simulink model "TwoQuadrantDCDCConverter"  (R2024a)
settings: Solver=VariableStepAuto  StartTime=0.0  StopTime=0.03  MaxStep=1e-4  RelTol=1e-4  EnableMultiTasking=on
libraries: spsGroundLib x3, spsDCVoltageSourceLib x2, spsSeriesRLCBranchLib x2, spsMeanLib x2, spsCurrentMeasurementLib x1, spsVoltageMeasurementLib x1, spsPWMGeneratorDCDCLib x1, spsTwoQuadrantDCDCConverterLib x1, sps_lib x1
settings Model: Creator=The MathWorks, Inc.  LastModifiedBy=nakamura
settings SolverCC: AlgebraicLoopSolver=TrustRegion  SolverResetMethod=Robust
settings OptimizationCC: LifeSpan=inf
settings DebuggingCC: ReadBeforeWriteMsg=DisableAll  WriteAfterWriteMsg=DisableAll  WriteAfterReadMsg=DisableAll  MultiTaskDSMMsg=none  UnconnectedInputMsg=warning  UnconnectedOutputMsg=warning  UnconnectedLineMsg=warning  SFUnexpectedBacktrackingDiag=warning  SFNoUnconditionalDefaultTransitionDiag=warning  SFExecutionAtInitializationDiag=none  ArithmeticOperatorsInVariantConditions=warning
settings ModelReferenceCC: UpdateModelReferenceTargets=IfOutOfDate  EnableRefExpFcnMdlSchedulingChecks=on
settings SFSimCC: SFSimEcho=off  SimUseLocalCustomCode=off  CustomCodeUndefinedFunction=UseInterfaceOnly
settings RTWCC: RTWUseLocalCustomCode=off  GPUComputeCapability=3.5
settings CodeAppCC: StateflowObjectComments=on
settings GRTTargetCC: TargetLangStandard=C89/C90 (ANSI)
settings ConfigComp: CovMetricSettings=dw  CovSaveCumulativeToWorkspaceVar=on  CovSaveSingleToWorkspaceVar=on  CovExternalEMLEnable=off
settings SimscapeCC: SimscapeNormalizeSystem=off  SimscapeNominalValues={1, 'bar'; 1, 'cm^3/s'; 1, 'bar*kg/s'; 1, 'kJ/kg'; 1, 'kW'; }

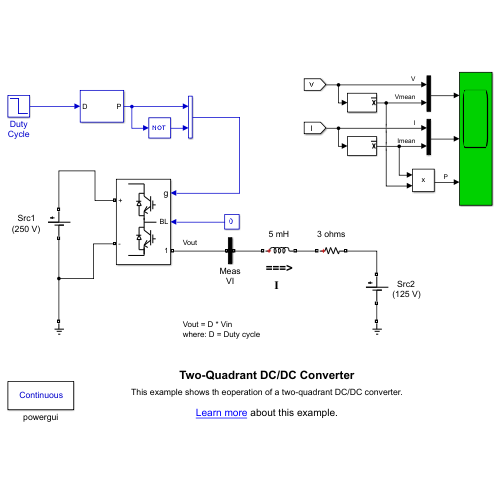
[thumbnail: Simulink's stored preview of the top-level diagram]
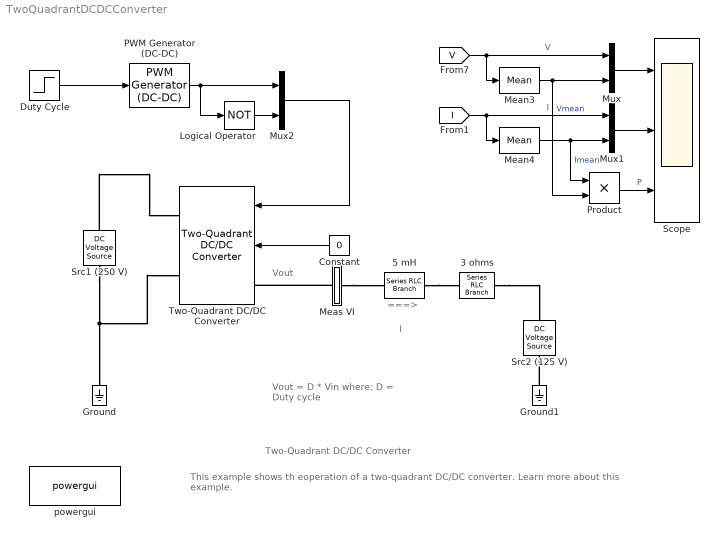
== system TwoQuadrantDCDCConverter ==
  note: Vout
  note: Vout = D * Vin
      | where: D = Duty cycle
  note: ===>
  note: I
  note: Two-Quadrant DC/DC Converter
  note: This example shows th eoperation of a two-quadrant DC/DC converter.
      |
      | Learn more about this example.
  "  Src2 (125 V)" : spsDCVoltageSourceLib/DC Voltage Source  Amplitude=125  Measurements=None
  3 ohms : spsSeriesRLCBranchLib/Series RLC Branch  LConnTagsString=__new0  RConnTagsString=__new0  BranchType=R  Resistance=3  Inductance=750e-6  SetiL0=on  InitialCurrent=14  Capacitance=30e-6  Setx0=off  InitialVoltage=150  Measurements=None
  5 mH : spsSeriesRLCBranchLib/Series RLC Branch  LConnTagsString=__new0  RConnTagsString=__new0  BranchType=L  Resistance=1e-4  Inductance=5e-3  SetiL0=off  InitialCurrent=14  Capacitance=30e-6  Setx0=off  InitialVoltage=150  Measurements=None
  Constant : Constant  Value=0
  Duty Cycle : Step  Time=0.015  Before=0.75  After=0.25  SampleTime=0
  Ground : spsGroundLib/Ground  LConnTagsString=a
  Ground1 : spsGroundLib/Ground  LConnTagsString=a
  Logical Operator : Logic  Operator=NOT  AllPortsSameDT=off  OutDataTypeStr=float('double')
  Mean3 : spsMeanLib/Mean  Freq=1000  Vinit=0  Ts=0
  Mean4 : spsMeanLib/Mean  Freq=1000  Vinit=0  Ts=0
  Meas VI : Subsystem
  Mux : Mux  Inputs=2
  Mux1 : Mux  Inputs=2
  Mux2 : Mux  Inputs=2
  PWM Generator (DC-DC) : spsPWMGeneratorDCDCLib/PWM Generator (DC-DC)  Fsw=2e3  Ts=0
  Product : Product
  Scope : Scope  NumInputPorts=3
  "Src1 (250 V) " : spsDCVoltageSourceLib/DC Voltage Source  Amplitude=250  Measurements=None
  Two-Quadrant DC/DC Converter : spsTwoQuadrantDCDCConverterLib/Two-Quadrant DC//DC Converter  ModelType=Switching devices  Ron=1e-3  Rs=1e6  Cs=inf  Vforward=[0,0]  Ron_Diode=1e-3  Rs_Diode=1e6  Cs_Diode=inf  Vf_Diode=1e-3  Rs_CurrentSource=inf  Ron_ACsource=1e-3
      settings: LibrarySourceBlock=|
      | sps_lib/Power Electronics/Two-Quadrant
      | DC//DC Converter
  powergui : sps_lib/powergui  Priority=1  SimulationMode=Continuous  SampleTime=1e-6  frequency=60  Iterations=50  frequencyindice=0  Pbase=100e6  ErrMax=1e-4  UnitsV=kV  UnitsW=MW  buscounter=0  FunctionMessages=off  echomessages=off  EnableUseOfTLC=off  CurrentSourceSwitches=off  DisableSnubberDevices=off  DisableRonSwitches=off  DisableVfSwitches=off  DisplayEquations=off  AutomaticDiscreteSolvers=off  SolverType=Tustin/Backward Euler (TBE)  Interpol=off  ExternalGateDelay=off  methode=off  Ts=100  x0status=blocks  SPID=on  SwTol=0  HookPort=off  NonlinearTolerance=1e-4  nMaxIteration=100  ContinueOnMaxIteration=off  RestoreLinks=warning  ResistiveCurrentMeasurement=off  Frange=[0:2:500]  Ylog=off  Xlog=on  ShowGrid=off  save=off  variable=ZData  structure=0  ZoomFFT=off  StartTime=0.0  cycles=1  DisplayStyle=1  fundamental=60  FreqAxis=off  MaxFrequency=1000  frequencyindicesteady=1  RmsSteady=1  display=off
  wires:
  Duty Cycle/1 -> PWM Generator (DC-DC)/1
  [V] -> Mean3/1, Mux/1  "V"
  Mux/1 -> Scope/1
  PWM Generator (DC-DC)/1 -> Logical Operator/1, Mux2/1
  Logical Operator/1 -> Mux2/2
  Constant/1 -> Two-Quadrant DC/DC Converter/2
  Mux2/1 -> Two-Quadrant DC/DC Converter/1
  Mean3/1 -> Product/2, Mux/2  "Vmean"
  [I] -> Mux1/1, Mean4/1  "I"
  Mean4/1 -> Product/1, Mux1/2  "Imean"
  Mux1/1 -> Scope/2
  Product/1 -> Scope/3  "P"
  connections:
  5 mH/RConn1 -- 3 ohms/LConn1
  3 ohms/RConn1 -- "  Src2 (125 V)"/RConn1
  "Src1 (250 V) "/RConn1 -- Two-Quadrant DC/DC Converter/RConn1
  "Src1 (250 V) "/LConn1 -- Two-Quadrant DC/DC Converter/RConn2 -- Ground/LConn1
  Meas VI/LConn1 -- Two-Quadrant DC/DC Converter/LConn1
  Meas VI/RConn1 -- 5 mH/LConn1
  Ground1/LConn1 -- "  Src2 (125 V)"/LConn1

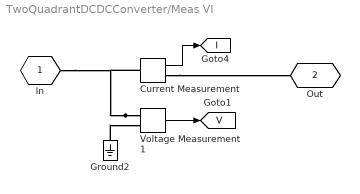
== system TwoQuadrantDCDCConverter/Meas VI ==
  Current Measurement : spsCurrentMeasurementLib/Current Measurement  PhasorSimulation=off  OutputType=Complex  PSBequivalent=0
  Ground2 : spsGroundLib/Ground  LConnTagsString=a
  Voltage Measurement1 : spsVoltageMeasurementLib/Voltage Measurement  Tag=PoWeRsYsTeMmEaSuReMeNt  PhasorSimulation=off  OutputType=Magnitude  PSBequivalent=0
  In : PMIOPort  Tag=PMCPort  Side=Left
  Out : PMIOPort  Tag=PMCPort  Port=2  Side=Right
  tag scope: I=global, V=global
  wires:
  Voltage Measurement1/1 -> [V]
  Current Measurement/1 -> [I]
  connections:
  Current Measurement/RConn1 -- Out/RConn1
  Voltage Measurement1/LConn1 -- Current Measurement/LConn1 -- In/RConn1
  Ground2/LConn1 -- Voltage Measurement1/LConn2
